simulink model "warp_timer"  (Simulink 7.1)
settings: Solver=ode45  StartTime=0.0  StopTime=1000  RelTol=1e-3
undefined symbols (not defined in the file): gcbh, xlBlockLoadCallback, xlGetSimulinkPeriod
libraries: xbsIndex_r4 x450
(part 2 of 5)

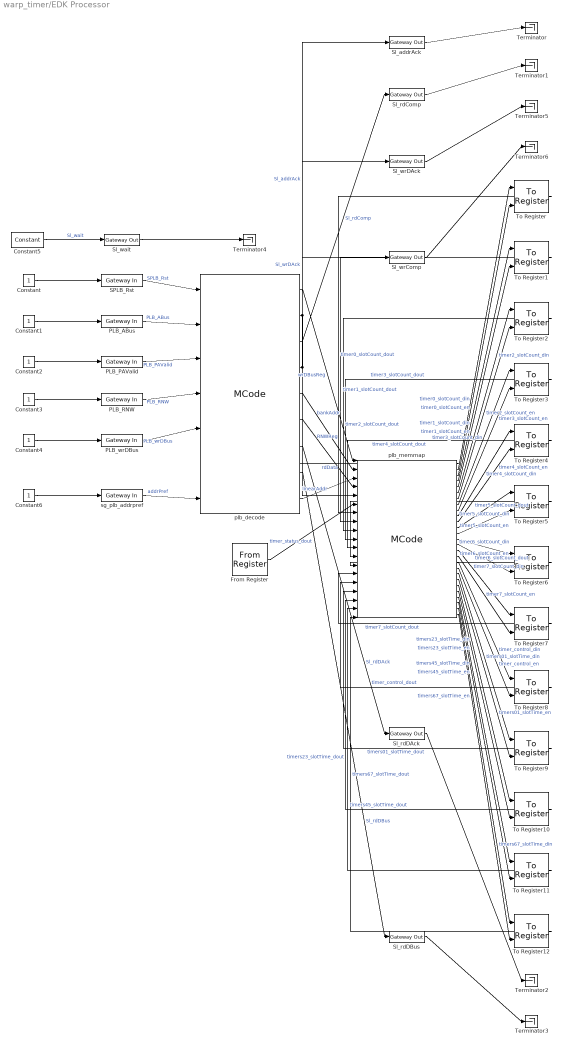
== system warp_timer/EDK Processor ==
  Constant{,1..4,6} (6 alike) : Constant
  Constant5 : xbsIndex_r4/Constant  arith_type=Unsigned  const=0  n_bits=1  bin_pt=0  explicit_period=on  period=xlGetSimulinkPeriod(gcb)  equ=P=C  opselect=C  inp2=PCIN>>17  opr=+  inp1=P  carry=CIN  dbl_ovrd=off  block_type=constant
  From Register : xbsIndex_r4/From Register  shared_memory_name='timer_status'  init=0  period=xlGetSimulinkPeriod(gcb)  ownership=Owned and initialized elsewhere  arith_type=Unsigned  n_bits=32  bin_pt=0  dbl_ovrd=off  block_type=fromreg
      settings: AttributesFormatString=<< %<shared_memory_name> >>  infoedit="Register block that reads data to a shared memory register.  Delay of one sample period."  block_version=10.1.3
  PLB_ABus : xbsIndex_r4/Gateway In  arith_type=Unsigned  n_bits=32  bin_pt=0  quantization="Round  (unbiased: +/- Inf)"  overflow=Saturate  period=xlGetSimulinkPeriod(gcb)  dbl_ovrd=off  timing_constraint=None  locs_specified=off  LOCs={}  block_type=gatewayin
      settings: infoedit="Gateway in block.  Converts inputs of type Simulink integer, double and fixed point to  Xilinx fixed point type.<P><P>Hardware notes:  In hardware these blocks become top level input ports."  sginterface={'Xilinx'=>{'jtaghwcosim'=>{'non_memory_mapped_port'=>'PLB_ABus'}},'iopad'=>{'constraint'=>'#'}}  block_version=10.1.3
  PLB_PAValid : xbsIndex_r4/Gateway In  arith_type=Unsigned  n_bits=1  bin_pt=0  quantization="Round  (unbiased: +/- Inf)"  overflow=Saturate  period=xlGetSimulinkPeriod(gcb)  dbl_ovrd=off  timing_constraint=None  locs_specified=off  LOCs={}  block_type=gatewayin
      settings: infoedit="Gateway in block.  Converts inputs of type Simulink integer, double and fixed point to  Xilinx fixed point type.<P><P>Hardware notes:  In hardware these blocks become top level input ports."  sginterface={'Xilinx'=>{'jtaghwcosim'=>{'non_memory_mapped_port'=>'PLB_PAValid'}},'iopad'=>{'constraint'=>'#'}}  block_version=10.1.3
  PLB_RNW : xbsIndex_r4/Gateway In  arith_type=Unsigned  n_bits=1  bin_pt=0  quantization="Round  (unbiased: +/- Inf)"  overflow=Saturate  period=xlGetSimulinkPeriod(gcb)  dbl_ovrd=off  timing_constraint=None  locs_specified=off  LOCs={}  block_type=gatewayin
      settings: infoedit="Gateway in block.  Converts inputs of type Simulink integer, double and fixed point to  Xilinx fixed point type.<P><P>Hardware notes:  In hardware these blocks become top level input ports."  sginterface={'Xilinx'=>{'jtaghwcosim'=>{'non_memory_mapped_port'=>'PLB_RNW'}},'iopad'=>{'constraint'=>'#'}}  block_version=10.1.3
  PLB_wrDBus : xbsIndex_r4/Gateway In  arith_type=Unsigned  n_bits=32  bin_pt=0  quantization="Round  (unbiased: +/- Inf)"  overflow=Saturate  period=xlGetSimulinkPeriod(gcb)  dbl_ovrd=off  timing_constraint=None  locs_specified=off  LOCs={}  block_type=gatewayin
      settings: infoedit="Gateway in block.  Converts inputs of type Simulink integer, double and fixed point to  Xilinx fixed point type.<P><P>Hardware notes:  In hardware these blocks become top level input ports."  sginterface={'Xilinx'=>{'jtaghwcosim'=>{'non_memory_mapped_port'=>'PLB_wrDBus'}},'iopad'=>{'constraint'=>'#'}}  block_version=10.1.3
  SPLB_Rst : xbsIndex_r4/Gateway In  arith_type=Unsigned  n_bits=1  bin_pt=0  quantization="Round  (unbiased: +/- Inf)"  overflow=Saturate  period=xlGetSimulinkPeriod(gcb)  dbl_ovrd=off  timing_constraint=None  locs_specified=off  LOCs={}  block_type=gatewayin
      settings: infoedit="Gateway in block.  Converts inputs of type Simulink integer, double and fixed point to  Xilinx fixed point type.<P><P>Hardware notes:  In hardware these blocks become top level input ports."  sginterface={'Xilinx'=>{'jtaghwcosim'=>{'non_memory_mapped_port'=>'SPLB_Rst'}},'iopad'=>{'constraint'=>'#'}}  block_version=10.1.3
  Sl_addrAck : xbsIndex_r4/Gateway Out  hdl_port=on  timing_constraint=None  locs_specified=off  LOCs={}  block_type=gatewayout
      settings: infoedit="Gateway out block.  Converts Xilinx fixed point inputs into ouputs of type Simulink integer, double, or fixed point.<P><P>Hardware notes:  In hardware these blocks become top level output ports or are discarded, depending on how they are configured."  sginterface={'Xilinx'=>{'jtaghwcosim'=>{'non_memory_mapped_port'=>'Sl_addrAck'}},'iopad'=>{'constraint'=>'#'}}  block_version=10.1.3
  Sl_rdComp : xbsIndex_r4/Gateway Out  hdl_port=on  timing_constraint=None  locs_specified=off  LOCs={}  block_type=gatewayout
      settings: infoedit="Gateway out block.  Converts Xilinx fixed point inputs into ouputs of type Simulink integer, double, or fixed point.<P><P>Hardware notes:  In hardware these blocks become top level output ports or are discarded, depending on how they are configured."  sginterface={'Xilinx'=>{'jtaghwcosim'=>{'non_memory_mapped_port'=>'Sl_rdComp'}},'iopad'=>{'constraint'=>'#'}}  block_version=10.1.3
  Sl_rdDAck : xbsIndex_r4/Gateway Out  hdl_port=on  timing_constraint=None  locs_specified=off  LOCs={}  block_type=gatewayout
      settings: infoedit="Gateway out block.  Converts Xilinx fixed point inputs into ouputs of type Simulink integer, double, or fixed point.<P><P>Hardware notes:  In hardware these blocks become top level output ports or are discarded, depending on how they are configured."  sginterface={'Xilinx'=>{'jtaghwcosim'=>{'non_memory_mapped_port'=>'Sl_rdDAck'}},'iopad'=>{'constraint'=>'#'}}  block_version=10.1.3
  Sl_rdDBus : xbsIndex_r4/Gateway Out  hdl_port=on  timing_constraint=None  locs_specified=off  LOCs={}  block_type=gatewayout
      settings: infoedit="Gateway out block.  Converts Xilinx fixed point inputs into ouputs of type Simulink integer, double, or fixed point.<P><P>Hardware notes:  In hardware these blocks become top level output ports or are discarded, depending on how they are configured."  sginterface={'Xilinx'=>{'jtaghwcosim'=>{'non_memory_mapped_port'=>'Sl_rdDBus'}},'iopad'=>{'constraint'=>'#'}}  block_version=10.1.3
  Sl_wait : xbsIndex_r4/Gateway Out  hdl_port=on  timing_constraint=None  locs_specified=off  LOCs={}  block_type=gatewayout
      settings: infoedit="Gateway out block.  Converts Xilinx fixed point inputs into ouputs of type Simulink integer, double, or fixed point.<P><P>Hardware notes:  In hardware these blocks become top level output ports or are discarded, depending on how they are configured."  sginterface={'Xilinx'=>{'jtaghwcosim'=>{'non_memory_mapped_port'=>'Sl_wait'}},'iopad'=>{'constraint'=>'#'}}  block_version=10.1.3
  Sl_wrComp : xbsIndex_r4/Gateway Out  hdl_port=on  timing_constraint=None  locs_specified=off  LOCs={}  block_type=gatewayout
      settings: infoedit="Gateway out block.  Converts Xilinx fixed point inputs into ouputs of type Simulink integer, double, or fixed point.<P><P>Hardware notes:  In hardware these blocks become top level output ports or are discarded, depending on how they are configured."  sginterface={'Xilinx'=>{'jtaghwcosim'=>{'non_memory_mapped_port'=>'Sl_wrComp'}},'iopad'=>{'constraint'=>'#'}}  block_version=10.1.3
  Sl_wrDAck : xbsIndex_r4/Gateway Out  hdl_port=on  timing_constraint=None  locs_specified=off  LOCs={}  block_type=gatewayout
      settings: infoedit="Gateway out block.  Converts Xilinx fixed point inputs into ouputs of type Simulink integer, double, or fixed point.<P><P>Hardware notes:  In hardware these blocks become top level output ports or are discarded, depending on how they are configured."  sginterface={'Xilinx'=>{'jtaghwcosim'=>{'non_memory_mapped_port'=>'Sl_wrDAck'}},'iopad'=>{'constraint'=>'#'}}  block_version=10.1.3
  Terminator{,1..6} (7 alike) : Terminator
  To Register : xbsIndex_r4/To Register  shared_memory_name='timer0_slotCount'  init=0  ownership=Owned and initialized elsewhere  explicit_data_type=on  arith_type=Unsigned  n_bits=32  bin_pt=0  dbl_ovrd=off  block_type=toreg
      settings: AttributesFormatString=<< %<shared_memory_name> >>  infoedit="Register block that writes data to a shared memory register.  Delay of one sample period."  block_version=10.1.3
  To Register1 : xbsIndex_r4/To Register  shared_memory_name='timer1_slotCount'  init=0  ownership=Owned and initialized elsewhere  explicit_data_type=on  arith_type=Unsigned  n_bits=32  bin_pt=0  dbl_ovrd=off  block_type=toreg
      settings: AttributesFormatString=<< %<shared_memory_name> >>  infoedit="Register block that writes data to a shared memory register.  Delay of one sample period."  block_version=10.1.3
  To Register10 : xbsIndex_r4/To Register  shared_memory_name='timers23_slotTime'  init=0  ownership=Owned and initialized elsewhere  explicit_data_type=on  arith_type=Unsigned  n_bits=32  bin_pt=0  dbl_ovrd=off  block_type=toreg
      settings: AttributesFormatString=<< %<shared_memory_name> >>  infoedit="Register block that writes data to a shared memory register.  Delay of one sample period."  block_version=10.1.3
  To Register11 : xbsIndex_r4/To Register  shared_memory_name='timers45_slotTime'  init=0  ownership=Owned and initialized elsewhere  explicit_data_type=on  arith_type=Unsigned  n_bits=32  bin_pt=0  dbl_ovrd=off  block_type=toreg
      settings: AttributesFormatString=<< %<shared_memory_name> >>  infoedit="Register block that writes data to a shared memory register.  Delay of one sample period."  block_version=10.1.3
  To Register12 : xbsIndex_r4/To Register  shared_memory_name='timers67_slotTime'  init=0  ownership=Owned and initialized elsewhere  explicit_data_type=on  arith_type=Unsigned  n_bits=32  bin_pt=0  dbl_ovrd=off  block_type=toreg
      settings: AttributesFormatString=<< %<shared_memory_name> >>  infoedit="Register block that writes data to a shared memory register.  Delay of one sample period."  block_version=10.1.3
  To Register2 : xbsIndex_r4/To Register  shared_memory_name='timer2_slotCount'  init=0  ownership=Owned and initialized elsewhere  explicit_data_type=on  arith_type=Unsigned  n_bits=32  bin_pt=0  dbl_ovrd=off  block_type=toreg
      settings: AttributesFormatString=<< %<shared_memory_name> >>  infoedit="Register block that writes data to a shared memory register.  Delay of one sample period."  block_version=10.1.3
  To Register3 : xbsIndex_r4/To Register  shared_memory_name='timer3_slotCount'  init=0  ownership=Owned and initialized elsewhere  explicit_data_type=on  arith_type=Unsigned  n_bits=32  bin_pt=0  dbl_ovrd=off  block_type=toreg
      settings: AttributesFormatString=<< %<shared_memory_name> >>  infoedit="Register block that writes data to a shared memory register.  Delay of one sample period."  block_version=10.1.3
  To Register4 : xbsIndex_r4/To Register  shared_memory_name='timer4_slotCount'  init=0  ownership=Owned and initialized elsewhere  explicit_data_type=on  arith_type=Unsigned  n_bits=32  bin_pt=0  dbl_ovrd=off  block_type=toreg
      settings: AttributesFormatString=<< %<shared_memory_name> >>  infoedit="Register block that writes data to a shared memory register.  Delay of one sample period."  block_version=10.1.3
  To Register5 : xbsIndex_r4/To Register  shared_memory_name='timer5_slotCount'  init=0  ownership=Owned and initialized elsewhere  explicit_data_type=on  arith_type=Unsigned  n_bits=32  bin_pt=0  dbl_ovrd=off  block_type=toreg
      settings: AttributesFormatString=<< %<shared_memory_name> >>  infoedit="Register block that writes data to a shared memory register.  Delay of one sample period."  block_version=10.1.3
  To Register6 : xbsIndex_r4/To Register  shared_memory_name='timer6_slotCount'  init=0  ownership=Owned and initialized elsewhere  explicit_data_type=on  arith_type=Unsigned  n_bits=32  bin_pt=0  dbl_ovrd=off  block_type=toreg
      settings: AttributesFormatString=<< %<shared_memory_name> >>  infoedit="Register block that writes data to a shared memory register.  Delay of one sample period."  block_version=10.1.3
  To Register7 : xbsIndex_r4/To Register  shared_memory_name='timer7_slotCount'  init=0  ownership=Owned and initialized elsewhere  explicit_data_type=on  arith_type=Unsigned  n_bits=32  bin_pt=0  dbl_ovrd=off  block_type=toreg
      settings: AttributesFormatString=<< %<shared_memory_name> >>  infoedit="Register block that writes data to a shared memory register.  Delay of one sample period."  block_version=10.1.3
  To Register8 : xbsIndex_r4/To Register  shared_memory_name='timer_control'  init=0  ownership=Owned and initialized elsewhere  explicit_data_type=on  arith_type=Unsigned  n_bits=32  bin_pt=0  dbl_ovrd=off  block_type=toreg
      settings: AttributesFormatString=<< %<shared_memory_name> >>  infoedit="Register block that writes data to a shared memory register.  Delay of one sample period."  block_version=10.1.3
  To Register9 : xbsIndex_r4/To Register  shared_memory_name='timers01_slotTime'  init=0  ownership=Owned and initialized elsewhere  explicit_data_type=on  arith_type=Unsigned  n_bits=32  bin_pt=0  dbl_ovrd=off  block_type=toreg
      settings: AttributesFormatString=<< %<shared_memory_name> >>  infoedit="Register block that writes data to a shared memory register.  Delay of one sample period."  block_version=10.1.3
  plb_decode : xbsIndex_r4/MCode  mfname=xlmax  explicit_period=off  period=1  dbl_ovrd=off  enable_stdout=off  enable_debug=off  mfilecontent=|  suppress_output=1  defparams={}  hide_port_list={}  block_type=mcode
      | function [wrDBusReg, addrAck, rdComp, wrDAck, bankAddr, RNWReg, rdDAck, rdDBus, linearAddr] = ...
      |     plb_bus_decode(plbRst, plbABus, plbPAValid, plbRNW, plbWrDBus, rdData, addrPref)
      | 
      | % constant variables (TODO: should pass from outside)
      | ADDRPREF_LEN = 20;
      | BANKADDR_LEN = 2;
      | LINEARADDR_LEN = 8;
      | ABUS_LEN = 32;
      | DBUS_LEN = 32;
      | 
      | % declare and initialize persistent variables
      | % register input bus signals
      | persistent plbRstReg_, plbRstReg_ = xl_state(0, {xlBoolean});
      | persistent plbABusReg_, plbABusReg_ = xl_state(0, {xlUnsigned, ABUS_LEN, 0});
      | persistent plbPAValidReg_, plbPAValidReg_ = xl_state(0, {xlBoolean});
      | persistent plbRNWReg_, plbRNWReg_ = xl_state(0, {xlUnsigned, 1, 0});
      | persistent plbWrDBusReg_, plbWrDBusReg_ = xl_state(0, {xlUnsigned, DBUS_LEN, 0});
      | 
      | % ===== rest of the outputs =====
      | 
      | bankAddr   = xl_slice(plbABusReg_, 2+BANKADDR_LEN+LINEARADDR_LEN-1, 2+LINEARADDR_LEN);
      | linearAddr = xl_slice(plbABusReg_, 2+LINEARADDR_LEN-1, 2);
      | RNWReg = plbRNWReg_;
      | wrDBusReg = plbWrDBusReg_;
      | 
      | % ===== p_select =====
      | 
      | % register PAValid
      | persistent aValidReg, aValidReg = xl_state(0, {xlBoolean});
      | aValidReg = plbPAValidReg_;
      | 
      | % extract and register the address prefix
      | addrPref_in = xl_slice(plbABusReg_, xl_nbits(plbABusReg_)-1, xl_nbits(plbABusReg_)-ADDRPREF_LEN);
      | if addrPref_in == addrPref
      |     ps1 = true;
      | else 
      |     ps1 = false;
      | end 
      | 
      | persistent ps1Reg, ps1Reg = xl_state(0, ps1);
      | ps1Reg = ps1;
      | 
      | ps = xl_and(ps1Reg, aValidReg);
      | 
      | % ===== addrAck =====
      | 
      | % register ps
      | persistent psReg, psReg = xl_state(0, ps);
      | 
      | addrAck = xfix({xlUnsigned, 1, 0}, xl_and(xl_not(plbRstReg_), ps, xl_not(psReg)));
      | 
      | psReg = ps;
      | 
      | % ===== rdComp, rd/wr DAck =====
      |  
      | rdComp1 = xfix({xlUnsigned, 1, 0}, xl_and(addrAck, RNWReg));
      | 
      | NUM_rdCompDelay = 3;
      | persistent rdCompDelay, rdCompDelay = xl_state(zeros(1, NUM_rdCompDelay), rdComp1, NUM_rdCompDelay);
      | rdComp2 = rdCompDelay.back;
      | rdCompDelay.push_front_pop_back(rdComp1);
      | 
      | persistent rdCompReg, rdCompReg = xl_state(0, rdComp1);
      | rdComp = rdCompReg;
      | rdCompReg = rdComp2;
      | 
      | persistent rdDAckReg, rdDAckReg = xl_state(0, rdComp1);
      | rdDAck = rdDAckReg;
      | rdDAckReg = rdComp;
      | 
      | persistent wrDAckReg, wrDAckReg = xl_state(0, addrAck);
      | wrDAck = wrDAckReg;
      | wrDAckReg = xl_and(addrAck, xl_not(RNWReg));
      | 
      | % ===== rdDBus =====
      | 
      | rdSel = xl_or(rdComp2, rdComp);
      | 
      | if rdSel == 1
      |     rdDBus1 = rdData;
      | else
      |     rdDBus1 = 0;
      | end % if
      | 
      | persistent rdDBusReg, rdDBusReg = xl_state(0, rdDBus1);
      | rdDBus = rdDBusReg;
      | rdDBusReg = rdDBus1;
      | 
      | % rdDBus = xl_concat(rdDBus32, rdDBus32);
      | % rdDBus = rdDBus32;
      | 
      | % ===== update the persistent variables =====
      | 
      | plbRstReg_ = plbRst;
      | plbABusReg_ = plbABus;
      | plbPAValidReg_ = plbPAValid;
      | plbRNWReg_ = plbRNW;
      | plbWrDBusReg_ = xl_slice(plbWrDBus, DBUS_LEN-1, 0);
      settings: block_version=10.1.3
  plb_memmap : xbsIndex_r4/MCode  mfname=xlmax  explicit_period=off  period=1  dbl_ovrd=off  enable_stdout=off  enable_debug=off  mfilecontent=|  suppress_output=1  defparams={}  hide_port_list={}  block_type=mcode
      | function [read_bank_out, sm_timer0_slotCount_din, sm_timer0_slotCount_en, sm_timer1_slotCount_din, sm_timer1_slotCount_en, sm_timer2_slotCount_din, sm_timer2_slotCount_en, sm_timer3_slotCount_din, sm_timer3_slotCount_en, sm_timer4_slotCount_din, sm_timer4_slotCount_en, sm_timer5_slotCount_din, sm_timer5_slotCount_en, sm_timer6_slotCount_din, sm_timer6_slotCount_en, sm_timer7_slotCount_din, sm_timer7_slotCount_en, sm_timer_control_din, sm_timer_control_en, sm_timers01_slotTime_din, sm_timers01_slotTime_en, sm_timers23_slotTime_din, sm_timers23_slotTime_en, sm_timers45_slotTime_din, sm_timers45_slotTime_en, sm_timers67_slotTime_din, sm_timers67_slotTime_en] = plb_memmap(wrDBus, bankAddr, linearAddr, RNWReg, addrAck, sm_timer_status, sm_timer0_slotCount, sm_timer1_slotCount, sm_timer2_slotCount, sm_timer3_slotCount, sm_timer4_slotCount, sm_timer5_slotCount, sm_timer6_slotCount, sm_timer7_slotCount, sm_timer_control, sm_timers01_slotTime, sm_timers23_slotTime, sm_timers45_slotTime, sm_timers67_slotTime)
      | 
      | 
      | % connvert the input data to UFix_32_0 (the bus data type)
      | % 'From Register' blocks
      | % sm_timer_status_bus = xfix({xlUnsigned, 32, 0}, 0);
      | sm_timer_status_bus = xl_force(sm_timer_status, xlUnsigned, 0);
      | 
      | % 'To Register' blocks
      | 
      | % sm_timer0_slotCount_dout = xfix({xlUnsigned, 32, 0}, 0);
      | sm_timer0_slotCount_dout = xl_force(sm_timer0_slotCount, xlUnsigned, 0);
      | 
      | % sm_timer1_slotCount_dout = xfix({xlUnsigned, 32, 0}, 0);
      | sm_timer1_slotCount_dout = xl_force(sm_timer1_slotCount, xlUnsigned, 0);
      | 
      | % sm_timer2_slotCount_dout = xfix({xlUnsigned, 32, 0}, 0);
      | sm_timer2_slotCount_dout = xl_force(sm_timer2_slotCount, xlUnsigned, 0);
      | 
      | % sm_timer3_slotCount_dout = xfix({xlUnsigned, 32, 0}, 0);
      | sm_timer3_slotCount_dout = xl_force(sm_timer3_slotCount, xlUnsigned, 0);
      | 
      | % sm_timer4_slotCount_dout = xfix({xlUnsigned, 32, 0}, 0);
      | sm_timer4_slotCount_dout = xl_force(sm_timer4_slotCount, xlUnsigned, 0);
      | 
      | % sm_timer5_slotCount_dout = xfix({xlUnsigned, 32, 0}, 0);
      | sm_timer5_slotCount_dout = xl_force(sm_timer5_slotCount, xlUnsigned, 0);
      | 
      | % sm_timer6_slotCount_dout = xfix({xlUnsigned, 32, 0}, 0);
      | sm_timer6_slotCount_dout = xl_force(sm_timer6_slotCount, xlUnsigned, 0);
      | 
      | % sm_timer7_slotCount_dout = xfix({xlUnsigned, 32, 0}, 0);
      | sm_timer7_slotCount_dout = xl_force(sm_timer7_slotCount, xlUnsigned, 0);
      | 
      | % sm_timer_control_dout = xfix({xlUnsigned, 32, 0}, 0);
      | sm_timer_control_dout = xl_force(sm_timer_control, xlUnsigned, 0);
      | 
      | % sm_timers01_slotTime_dout = xfix({xlUnsigned, 32, 0}, 0);
      | sm_timers01_slotTime_dout = xl_force(sm_timers01_slotTime, xlUnsigned, 0);
      | 
      | % sm_timers23_slotTime_dout = xfix({xlUnsigned, 32, 0}, 0);
      | sm_timers23_slotTime_dout = xl_force(sm_timers23_slotTime, xlUnsigned, 0);
      | 
      | % sm_timers45_slotTime_dout = xfix({xlUnsigned, 32, 0}, 0);
      | sm_timers45_slotTime_dout = xl_force(sm_timers45_slotTime, xlUnsigned, 0);
      | 
      | % sm_timers67_slotTime_dout = xfix({xlUnsigned, 32, 0}, 0);
      | sm_timers67_slotTime_dout = xl_force(sm_timers67_slotTime, xlUnsigned, 0);
      | 
      | 
      | % 'From FIFO' blocks
      | % 'To FIFO' blocks
      | % 'Shared Memory' blocks
      | 
      | % 'dout' ports of 'From Register' blocks
      | 
      | % registered register mux output
      | persistent reg_bank_out_reg; reg_bank_out_reg = xl_state(0, {xlUnsigned, 32, 0});
      | reg_bank_out = reg_bank_out_reg;
      | 
      | if linearAddr == 13
      |     reg_bank_out_reg = sm_timer_status_bus;
      | elseif linearAddr == 0
      |     reg_bank_out_reg = sm_timer0_slotCount_dout;
      | elseif linearAddr == 1
      |     reg_bank_out_reg = sm_timer1_slotCount_dout;
      | elseif linearAddr == 2
      |     reg_bank_out_reg = sm_timer2_slotCount_dout;
      | elseif linearAddr == 3
      |     reg_bank_out_reg = sm_timer3_slotCount_dout;
      | elseif linearAddr == 4
      |     reg_bank_out_reg = sm_timer4_slotCount_dout;
      | elseif linearAddr == 5
      |     reg_bank_out_reg = sm_timer5_slotCount_dout;
      | elseif linearAddr == 6
      |     reg_bank_out_reg = sm_timer6_slotCount_dout;
      | elseif linearAddr == 7
      |     reg_bank_out_reg = sm_timer7_slotCount_dout;
      | elseif linearAddr == 8
      |     reg_bank_out_reg = sm_timer_control_dout;
      | elseif linearAddr == 9
      |     reg_bank_out_reg = sm_timers01_slotTime_dout;
      | elseif linearAddr == 10
      |     reg_bank_out_reg = sm_timers23_slotTime_dout;
      | elseif linearAddr == 11
      |     reg_bank_out_reg = sm_timers45_slotTime_dout;
      | elseif linearAddr == 12
      |     reg_bank_out_reg = sm_timers67_slotTime_dout;
      | 
      | end
      | 
      | 
      | % 'From FIFO' and 'To FIFO' blocks
      | 
      | 
      | 
      | 
      | 
      | opCode = xl_concat(addrAck, RNWReg, bankAddr, linearAddr);
      | 
      | % 'Shared Memory' blocks
      | 
      | 
      | 
      | 
      | 
      | % 'din' ports of 'Shared Memory' blocks
      | 
      | 
      | % 'we' ports of 'Shared Memory' blocks
      | 
      | 
      | % 'addr' ports of 'Shared Memory' blocks
      | 
      | 
      | % 're' ports of 'From FIFO' blocks
      | 
      | 
      | % 'en' ports of 'To Register' blocks
      | if opCode == xl_concat(xfix({xlUnsigned, 4, 0}, 10), ...
      |                        xfix({xlUnsigned, xl_nbits(linearAddr), 0}, 0))
      |     sm_timer0_slotCount_en = true;
      | else
      |     sm_timer0_slotCount_en = false;
      | end
      | if opCode == xl_concat(xfix({xlUnsigned, 4, 0}, 10), ...
      |                        xfix({xlUnsigned, xl_nbits(linearAddr), 0}, 1))
      |     sm_timer1_slotCount_en = true;
      | else
      |     sm_timer1_slotCount_en = false;
      | end
      | if opCode == xl_concat(xfix({xlUnsigned, 4, 0}, 10), ...
      |                        xfix({xlUnsigned, xl_nbits(linearAddr), 0}, 2))
      |     sm_timer2_slotCount_en = true;
      | else
      |     sm_timer2_slotCount_en = false;
      | end
      | if opCode == xl_concat(xfix({xlUnsigned, 4, 0}, 10), ...
      |                        xfix({xlUnsigned, xl_nbits(linearAddr), 0}, 3))
      |     sm_timer3_slotCount_en = true;
      | else
      |     sm_timer3_slotCount_en = false;
      | end
      | if opCode == xl_concat(xfix({xlUnsigned, 4, 0}, 10), ...
      |                        xfix({xlUnsigned, xl_nbits(linearAddr), 0}, 4))
      |     sm_timer4_slotCount_en = true;
      | else
      |     sm_timer4_slotCount_en = false;
      | end
      | if opCode == xl_concat(xfix({xlUnsigned, 4, 0}, 10), ...
      |                        xfix({xlUnsigned, xl_nbits(linearAddr), 0}, 5))
      |     sm_timer5_slotCount_en = true;
      | else
      |     sm_timer5_slotCount_en = false;
      | end
      | if opCode == xl_concat(xfix({xlUnsigned, 4, 0}, 10), ...
      |                        xfix({xlUnsigned, xl_nbits(linearAddr), 0}, 6))
      |     sm_timer6_slotCount_en = true;
      | else
      |     sm_timer6_slotCount_en = false;
      | end
      | if opCode == xl_concat(xfix({xlUnsigned, 4, 0}, 10), ...
      |                        xfix({xlUnsigned, xl_nbits(linearAddr), 0}, 7))
      |     sm_timer7_slotCount_en = true;
      | else
      |     sm_timer7_slotCount_en = false;
      | end
      | if opCode == xl_concat(xfix({xlUnsigned, 4, 0}, 10), ...
      |                        xfix({xlUnsigned, xl_nbits(linearAddr), 0}, 8))
      |     sm_timer_control_en = true;
      | else
      |     sm_timer_control_en = false;
      | end
      | if opCode == xl_concat(xfix({xlUnsigned, 4, 0}, 10), ...
      |                        xfix({xlUnsigned, xl_nbits(linearAddr), 0}, 9))
      |     sm_timers01_slotTime_en = true;
      | else
      |     sm_timers01_slotTime_en = false;
      | end
      | if opCode == xl_concat(xfix({xlUnsigned, 4, 0}, 10), ...
      |                        xfix({xlUnsigned, xl_nbits(linearAddr), 0}, 10))
      |     sm_timers23_slotTime_en = true;
      | else
      |     sm_timers23_slotTime_en = false;
      | end
      | if opCode == xl_concat(xfix({xlUnsigned, 4, 0}, 10), ...
      |                        xfix({xlUnsigned, xl_nbits(linearAddr), 0}, 11))
      |     sm_timers45_slotTime_en = true;
      | else
      |     sm_timers45_slotTime_en = false;
      | end
      | if opCode == xl_concat(xfix({xlUnsigned, 4, 0}, 10), ...
      |                        xfix({xlUnsigned, xl_nbits(linearAddr), 0}, 12))
      |     sm_timers67_slotTime_en = true;
      | else
      |     sm_timers67_slotTime_en = false;
      | end
      | 
      | 
      | % 'din' ports of 'To FIFO' blocks
      | 
      | 
      | % 'we' ports of 'To FIFO' blocks
      | 
      | 
      | % 'din' ports of 'To Register' blocks
      | sm_timer0_slotCount_din = xl_force(xl_slice(wrDBus, 32 - 1, 0), ...
      |                                  xlUnsigned, ...
      |                                  0);
      | sm_timer1_slotCount_din = xl_force(xl_slice(wrDBus, 32 - 1, 0), ...
      |                                  xlUnsigned, ...
      |                                  0);
      | sm_timer2_slotCount_din = xl_force(xl_slice(wrDBus, 32 - 1, 0), ...
      |                                  xlUnsigned, ...
      |                                  0);
      | sm_timer3_slotCount_din = xl_force(xl_slice(wrDBus, 32 - 1, 0), ...
      |                                  xlUnsigned, ...
      |                                  0);
      | sm_timer4_slotCount_din = xl_force(xl_slice(wrDBus, 32 - 1, 0), ...
      |                                  xlUnsigned, ...
      |                                  0);
      | sm_timer5_slotCount_din = xl_force(xl_slice(wrDBus, 32 - 1, 0), ...
      |                                  xlUnsigned, ...
      |                                  0);
      | sm_timer6_slotCount_din = xl_force(xl_slice(wrDBus, 32 - 1, 0), ...
      |                                  xlUnsigned, ...
      |                                  0);
      | sm_timer7_slotCount_din = xl_force(xl_slice(wrDBus, 32 - 1, 0), ...
      |                                  xlUnsigned, ...
      |                                  0);
      | sm_timer_control_din = xl_force(xl_slice(wrDBus, 32 - 1, 0), ...
      |                                  xlUnsigned, ...
      |                                  0);
      | sm_timers01_slotTime_din = xl_force(xl_slice(wrDBus, 32 - 1, 0), ...
      |                                  xlUnsigned, ...
      |                                  0);
      | sm_timers23_slotTime_din = xl_force(xl_slice(wrDBus, 32 - 1, 0), ...
      |                                  xlUnsigned, ...
      |                                  0);
      | sm_timers45_slotTime_din = xl_force(xl_slice(wrDBus, 32 - 1, 0), ...
      |                                  xlUnsigned, ...
      |                                  0);
      | sm_timers67_slotTime_din = xl_force(xl_slice(wrDBus, 32 - 1, 0), ...
      |                                  xlUnsigned, ...
      |                                  0);
      | 
      | 
      | persistent read_bank_out_reg; read_bank_out_reg = xl_state(0, {xlUnsigned, 32, 0});
      | read_bank_out = read_bank_out_reg;
      | 
      | persistent bankAddr_reg; bankAddr_reg = xl_state(0, bankAddr);
      | 
      | if bankAddr_reg == 0
      |     % Bank 0: Shared Memories
      |     read_bank_out_reg = 0;
      | elseif bankAddr_reg == 1
      |     % Bank 1: From/To FIFOs
      |     read_bank_out_reg =  0;
      | elseif bankAddr_reg == 2
      |     % Bank 2: From/To Registers
      |     read_bank_out_reg = reg_bank_out;
      | elseif bankAddr_reg == 3
      |     % Bank 3: Configuration Registers
      |     read_bank_out_reg = 0;
      | end
      | 
      | bankAddr_reg = bankAddr;
      settings: block_version=10.1.3
  sg_plb_addrpref : xbsIndex_r4/Gateway In  arith_type=Unsigned  n_bits=20  bin_pt=0  quantization="Round  (unbiased: +/- Inf)"  overflow=Saturate  period=xlGetSimulinkPeriod(gcb)  dbl_ovrd=off  timing_constraint=None  locs_specified=off  LOCs={}  block_type=gatewayin
      settings: infoedit="Gateway in block.  Converts inputs of type Simulink integer, double and fixed point to  Xilinx fixed point type.<P><P>Hardware notes:  In hardware these blocks become top level input ports."  sginterface={'Xilinx'=>{'jtaghwcosim'=>{'non_memory_mapped_port'=>'sg_plb_addrpref'}},'iopad'=>{'constraint'=>'#'}}  block_version=10.1.3
  wires:
  plb_decode/2 -> plb_memmap/5, Sl_addrAck/1  "Sl_addrAck"
  plb_decode/4 -> Sl_wrDAck/1, Sl_wrComp/1  "Sl_wrDAck"
  plb_memmap/27 -> To Register12/2  "timers67_slotTime_en"
  plb_memmap/26 -> To Register12/1  "timers67_slotTime_din"
  plb_memmap/25 -> To Register11/2  "timers45_slotTime_en"
  plb_memmap/24 -> To Register11/1  "timers45_slotTime_din"
  plb_memmap/23 -> To Register10/2  "timers23_slotTime_en"
  plb_memmap/22 -> To Register10/1  "timers23_slotTime_din"
  plb_memmap/21 -> To Register9/2  "timers01_slotTime_en"
  plb_memmap/20 -> To Register9/1  "timers01_slotTime_din"
  plb_memmap/19 -> To Register8/2  "timer_control_en"
  plb_memmap/18 -> To Register8/1  "timer_control_din"
  plb_memmap/17 -> To Register7/2  "timer7_slotCount_en"
  plb_memmap/16 -> To Register7/1  "timer7_slotCount_din"
  plb_memmap/15 -> To Register6/2  "timer6_slotCount_en"
  plb_memmap/14 -> To Register6/1  "timer6_slotCount_din"
  plb_memmap/13 -> To Register5/2  "timer5_slotCount_en"
  plb_memmap/12 -> To Register5/1  "timer5_slotCount_din"
  plb_memmap/11 -> To Register4/2  "timer4_slotCount_en"
  plb_memmap/10 -> To Register4/1  "timer4_slotCount_din"
  plb_memmap/9 -> To Register3/2  "timer3_slotCount_en"
  plb_memmap/8 -> To Register3/1  "timer3_slotCount_din"
  plb_memmap/7 -> To Register2/2  "timer2_slotCount_en"
  plb_memmap/6 -> To Register2/1  "timer2_slotCount_din"
  plb_memmap/5 -> To Register1/2  "timer1_slotCount_en"
  plb_memmap/4 -> To Register1/1  "timer1_slotCount_din"
  plb_memmap/3 -> To Register/2  "timer0_slotCount_en"
  plb_memmap/2 -> To Register/1  "timer0_slotCount_din"
  plb_memmap/1 -> plb_decode/6  "rdData"
  To Register12/1 -> plb_memmap/19  "timers67_slotTime_dout"
  To Register11/1 -> plb_memmap/18  "timers45_slotTime_dout"
  To Register10/1 -> plb_memmap/17  "timers23_slotTime_dout"
  To Register9/1 -> plb_memmap/16  "timers01_slotTime_dout"
  To Register8/1 -> plb_memmap/15  "timer_control_dout"
  To Register7/1 -> plb_memmap/14  "timer7_slotCount_dout"
  To Register6/1 -> plb_memmap/13  "timer6_slotCount_dout"
  To Register5/1 -> plb_memmap/12  "timer5_slotCount_dout"
  To Register4/1 -> plb_memmap/11  "timer4_slotCount_dout"
  To Register3/1 -> plb_memmap/10  "timer3_slotCount_dout"
  To Register2/1 -> plb_memmap/9  "timer2_slotCount_dout"
  To Register1/1 -> plb_memmap/8  "timer1_slotCount_dout"
  To Register/1 -> plb_memmap/7  "timer0_slotCount_dout"
  From Register/1 -> plb_memmap/6  "timer_status_dout"
  plb_decode/6 -> plb_memmap/4  "RNWReg"
  plb_decode/9 -> plb_memmap/3  "linearAddr"
  plb_decode/5 -> plb_memmap/2  "bankAddr"
  plb_decode/1 -> plb_memmap/1  "wrDBusReg"
  plb_decode/8 -> Sl_rdDBus/1  "Sl_rdDBus"
  plb_decode/7 -> Sl_rdDAck/1  "Sl_rdDAck"
  plb_decode/3 -> Sl_rdComp/1  "Sl_rdComp"
  sg_plb_addrpref/1 -> plb_decode/7  "addrPref"
  PLB_wrDBus/1 -> plb_decode/5  "PLB_wrDBus"
  PLB_RNW/1 -> plb_decode/4  "PLB_RNW"
  PLB_PAValid/1 -> plb_decode/3  "PLB_PAValid"
  PLB_ABus/1 -> plb_decode/2  "PLB_ABus"
  SPLB_Rst/1 -> plb_decode/1  "SPLB_Rst"
  Constant6/1 -> sg_plb_addrpref/1
  Constant5/1 -> Sl_wait/1  "Sl_wait"
  Constant4/1 -> PLB_wrDBus/1
  Constant3/1 -> PLB_RNW/1
  Constant2/1 -> PLB_PAValid/1
  Constant1/1 -> PLB_ABus/1
  Constant/1 -> SPLB_Rst/1
  Sl_wrComp/1 -> Terminator6/1
  Sl_wrDAck/1 -> Terminator5/1
  Sl_wait/1 -> Terminator4/1
  Sl_rdDBus/1 -> Terminator3/1
  Sl_rdDAck/1 -> Terminator2/1
  Sl_rdComp/1 -> Terminator1/1
  Sl_addrAck/1 -> Terminator/1

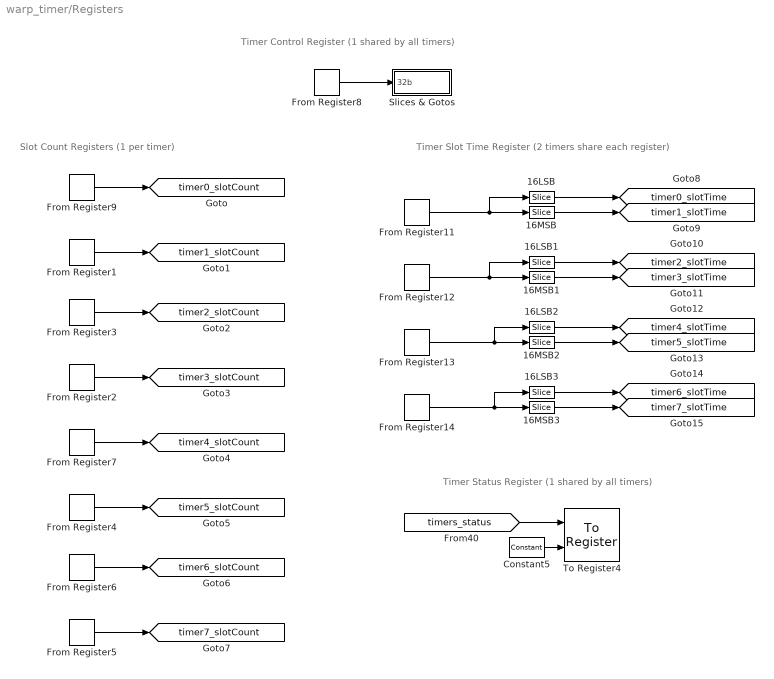
== system warp_timer/Registers ==
  note: Slot Count Registers
      | (1 per timer)
  note: Timer Control Register
      | (1 shared by all timers)
  note: Timer Slot Time Register
      | (2 timers share each register)
  note: Timer Status Register
      | (1 shared by all timers)
  16LSB{,1..3} (4 alike) : xbsIndex_r4/Slice  nbits=16  boolean_output=off  mode=Lower Bit Location + Width  bit1=0  base1=LSB of Input  bit0=0  base0=LSB of Input  dbl_ovrd=off  block_type=slice
      settings: infoedit="Extracts a given range of bits from each input sample and presents it at the output.  The output type is ordinarily unsigned with binary point at zero, but can be Boolean when the slice is one bit wide.<P><P>Hardware notes: In hardware this block costs nothing."  block_version=9.1.01
  16MSB{,1..3} (4 alike) : xbsIndex_r4/Slice  nbits=16  boolean_output=off  mode=Lower Bit Location + Width  bit1=0  base1=LSB of Input  bit0=16  base0=LSB of Input  dbl_ovrd=off  block_type=slice
      settings: infoedit="Extracts a given range of bits from each input sample and presents it at the output.  The output type is ordinarily unsigned with binary point at zero, but can be Boolean when the slice is one bit wide.<P><P>Hardware notes: In hardware this block costs nothing."  block_version=9.1.01
  Constant5 : xbsIndex_r4/Constant  arith_type=Boolean  const=1  n_bits=1  bin_pt=0  explicit_period=off  period=1  equ=P=C  opselect=C  inp2=PCIN>>17  opr=+  inp1=P  carry=CIN  dbl_ovrd=off  block_type=constant
      settings: block_version=8.2
  From Register1 : xbsIndex_r4/From Register  shared_memory_name='timer1_slotCount'  init=500  period=1  ownership=Locally owned and initialized  arith_type=Unsigned  n_bits=32  bin_pt=0  dbl_ovrd=off  block_type=fromreg
      settings: AttributesFormatString=From Register\n<< %<shared_memory_name> >>  infoedit="Register block that reads data to a shared memory register.  Delay of one sample period."  block_version=8.2
  From Register11 : xbsIndex_r4/From Register  shared_memory_name='timers01_slotTime'  init=0  period=1  ownership=Locally owned and initialized  arith_type=Unsigned  n_bits=32  bin_pt=0  dbl_ovrd=off  block_type=fromreg
      settings: AttributesFormatString=From Register\n<< %<shared_memory_name> >>  infoedit="Register block that reads data to a shared memory register.  Delay of one sample period."  block_version=8.2
  From Register12 : xbsIndex_r4/From Register  shared_memory_name='timers23_slotTime'  init=0  period=1  ownership=Locally owned and initialized  arith_type=Unsigned  n_bits=32  bin_pt=0  dbl_ovrd=off  block_type=fromreg
      settings: AttributesFormatString=From Register\n<< %<shared_memory_name> >>  infoedit="Register block that reads data to a shared memory register.  Delay of one sample period."  block_version=8.2
  From Register13 : xbsIndex_r4/From Register  shared_memory_name='timers45_slotTime'  init=0  period=1  ownership=Locally owned and initialized  arith_type=Unsigned  n_bits=32  bin_pt=0  dbl_ovrd=off  block_type=fromreg
      settings: AttributesFormatString=From Register\n<< %<shared_memory_name> >>  infoedit="Register block that reads data to a shared memory register.  Delay of one sample period."  block_version=8.2
  From Register14 : xbsIndex_r4/From Register  shared_memory_name='timers67_slotTime'  init=0  period=1  ownership=Locally owned and initialized  arith_type=Unsigned  n_bits=32  bin_pt=0  dbl_ovrd=off  block_type=fromreg
      settings: AttributesFormatString=From Register\n<< %<shared_memory_name> >>  infoedit="Register block that reads data to a shared memory register.  Delay of one sample period."  block_version=8.2
  From Register2 : xbsIndex_r4/From Register  shared_memory_name='timer3_slotCount'  init=500  period=1  ownership=Locally owned and initialized  arith_type=Unsigned  n_bits=32  bin_pt=0  dbl_ovrd=off  block_type=fromreg
      settings: AttributesFormatString=From Register\n<< %<shared_memory_name> >>  infoedit="Register block that reads data to a shared memory register.  Delay of one sample period."  block_version=8.2
  From Register3 : xbsIndex_r4/From Register  shared_memory_name='timer2_slotCount'  init=500  period=1  ownership=Locally owned and initialized  arith_type=Unsigned  n_bits=32  bin_pt=0  dbl_ovrd=off  block_type=fromreg
      settings: AttributesFormatString=From Register\n<< %<shared_memory_name> >>  infoedit="Register block that reads data to a shared memory register.  Delay of one sample period."  block_version=8.2
  From Register4 : xbsIndex_r4/From Register  shared_memory_name='timer5_slotCount'  init=500  period=1  ownership=Locally owned and initialized  arith_type=Unsigned  n_bits=32  bin_pt=0  dbl_ovrd=off  block_type=fromreg
      settings: AttributesFormatString=From Register\n<< %<shared_memory_name> >>  infoedit="Register block that reads data to a shared memory register.  Delay of one sample period."  block_version=8.2
  From Register5 : xbsIndex_r4/From Register  shared_memory_name='timer7_slotCount'  init=500  period=1  ownership=Locally owned and initialized  arith_type=Unsigned  n_bits=32  bin_pt=0  dbl_ovrd=off  block_type=fromreg
      settings: AttributesFormatString=From Register\n<< %<shared_memory_name> >>  infoedit="Register block that reads data to a shared memory register.  Delay of one sample period."  block_version=8.2
  From Register6 : xbsIndex_r4/From Register  shared_memory_name='timer6_slotCount'  init=500  period=1  ownership=Locally owned and initialized  arith_type=Unsigned  n_bits=32  bin_pt=0  dbl_ovrd=off  block_type=fromreg
      settings: AttributesFormatString=From Register\n<< %<shared_memory_name> >>  infoedit="Register block that reads data to a shared memory register.  Delay of one sample period."  block_version=8.2
  From Register7 : xbsIndex_r4/From Register  shared_memory_name='timer4_slotCount'  init=500  period=1  ownership=Locally owned and initialized  arith_type=Unsigned  n_bits=32  bin_pt=0  dbl_ovrd=off  block_type=fromreg
      settings: AttributesFormatString=From Register\n<< %<shared_memory_name> >>  infoedit="Register block that reads data to a shared memory register.  Delay of one sample period."  block_version=8.2
  From Register8 : xbsIndex_r4/From Register  shared_memory_name='timer_control'  init=0  period=1  ownership=Locally owned and initialized  arith_type=Unsigned  n_bits=32  bin_pt=0  dbl_ovrd=off  block_type=fromreg
      settings: AttributesFormatString=From Register\n<< %<shared_memory_name> >>  infoedit="Register block that reads data to a shared memory register.  Delay of one sample period."  block_version=8.2
  From Register9 : xbsIndex_r4/From Register  shared_memory_name='timer0_slotCount'  init=500  period=1  ownership=Locally owned and initialized  arith_type=Unsigned  n_bits=32  bin_pt=0  dbl_ovrd=off  block_type=fromreg
      settings: AttributesFormatString=From Register\n<< %<shared_memory_name> >>  infoedit="Register block that reads data to a shared memory register.  Delay of one sample period."  block_version=8.2
  Slices & Gotos : Subsystem
  To Register4 : xbsIndex_r4/To Register  shared_memory_name='timer_status'  init=0  ownership=Locally owned and initialized  explicit_data_type=on  arith_type=Unsigned  n_bits=32  bin_pt=0  dbl_ovrd=off  block_type=toreg
      settings: AttributesFormatString=To Register\n<< %<shared_memory_name> >>  infoedit="Register block that writes data to a shared memory register.  Delay of one sample period."  block_version=9.1.01
  tag scope: timer0_slotCount=global, timer0_slotTime=global, timer1_slotCount=global, timer1_slotTime=global, timer2_slotCount=global, timer2_slotTime=global, timer3_slotCount=global, timer3_slotTime=global, timer4_slotCount=global, timer4_slotTime=global, timer5_slotCount=global, timer5_slotTime=global, timer6_slotCount=global, timer6_slotTime=global, timer7_slotCount=global, timer7_slotTime=global
  wires:
  From Register8/1 -> Slices & Gotos/1(32b)
  From Register9/1 -> [timer0_slotCount]
  From Register5/1 -> [timer7_slotCount]
  From Register6/1 -> [timer6_slotCount]
  From Register4/1 -> [timer5_slotCount]
  From Register7/1 -> [timer4_slotCount]
  From Register2/1 -> [timer3_slotCount]
  From Register3/1 -> [timer2_slotCount]
  From Register1/1 -> [timer1_slotCount]
  From Register11/1 -> 16MSB/1, 16LSB/1
  16LSB/1 -> [timer0_slotTime]
  16MSB/1 -> [timer1_slotTime]
  16LSB1/1 -> [timer2_slotTime]
  16MSB1/1 -> [timer3_slotTime]
  16LSB2/1 -> [timer4_slotTime]
  16MSB2/1 -> [timer5_slotTime]
  16LSB3/1 -> [timer6_slotTime]
  16MSB3/1 -> [timer7_slotTime]
  From Register12/1 -> 16LSB1/1, 16MSB1/1
  From Register13/1 -> 16LSB2/1, 16MSB2/1
  From Register14/1 -> 16LSB3/1, 16MSB3/1
  Constant5/1 -> To Register4/2
  [timers_status] -> To Register4/1

== system warp_timer/Status Outputs ==
  T0 : Inport
  T1 : Inport  Port=2
  T2 : Inport  Port=3
  T3 : Inport  Port=4
  T4 : Inport  Port=5
  T5 : Inport  Port=6
  T6 : Inport  Port=7
  T7 : Inport  Port=8
  Concat13 : xbsIndex_r4/Concat  num_inputs=8  dbl_ovrd=off  block_type=concat
      settings: block_version=9.1.01
  LSB+{1..8} (8 alike) : xbsIndex_r4/Slice  nbits=1  boolean_output=off  mode=Lower Bit Location + Width  bit1=0  base1=LSB of Input  bit0=1  base0=LSB of Input  dbl_ovrd=off  block_type=slice
      settings: infoedit="Extracts a given range of bits from each input sample and presents it at the output.  The output type is ordinarily unsigned with binary point at zero, but can be Boolean when the slice is one bit wide.<P><P>Hardware notes: In hardware this block costs nothing."  block_version=9.1.01
  Logical : xbsIndex_r4/Logical  logical_function=OR  inputs=8  en=off  latency=0  precision=Full  arith_type=Unsigned  n_bits=16  bin_pt=0  align_bp=on  dbl_ovrd=off  block_type=logical
  TIMEREXPIRE : xbsIndex_r4/Gateway Out  hdl_port=on  timing_constraint=None  locs_specified=off  LOCs={}  block_type=gatewayout
      settings: infoedit="Gateway out block.  Converts Xilinx fixed point inputs into ouputs of type Simulink integer, double, or fixed point.<P><P>Hardware notes:  In hardware these blocks become top level output ports or are discarded, depending on how they are configured."  block_version=8.2
  timer0_active : xbsIndex_r4/Gateway Out  hdl_port=on  timing_constraint=None  locs_specified=off  LOCs={}  block_type=gatewayout
      settings: infoedit="Gateway out block.  Converts Xilinx fixed point inputs into ouputs of type Simulink integer, double, or fixed point.<P><P>Hardware notes:  In hardware these blocks become top level output ports or are discarded, depending on how they are configured."
  timer1_active : xbsIndex_r4/Gateway Out  hdl_port=on  timing_constraint=None  locs_specified=off  LOCs={}  block_type=gatewayout
      settings: infoedit="Gateway out block.  Converts Xilinx fixed point inputs into ouputs of type Simulink integer, double, or fixed point.<P><P>Hardware notes:  In hardware these blocks become top level output ports or are discarded, depending on how they are configured."
  timer2_active : xbsIndex_r4/Gateway Out  hdl_port=on  timing_constraint=None  locs_specified=off  LOCs={}  block_type=gatewayout
      settings: infoedit="Gateway out block.  Converts Xilinx fixed point inputs into ouputs of type Simulink integer, double, or fixed point.<P><P>Hardware notes:  In hardware these blocks become top level output ports or are discarded, depending on how they are configured."
  timer3_active : xbsIndex_r4/Gateway Out  hdl_port=on  timing_constraint=None  locs_specified=off  LOCs={}  block_type=gatewayout
      settings: infoedit="Gateway out block.  Converts Xilinx fixed point inputs into ouputs of type Simulink integer, double, or fixed point.<P><P>Hardware notes:  In hardware these blocks become top level output ports or are discarded, depending on how they are configured."
  timer4_active : xbsIndex_r4/Gateway Out  hdl_port=on  timing_constraint=None  locs_specified=off  LOCs={}  block_type=gatewayout
      settings: infoedit="Gateway out block.  Converts Xilinx fixed point inputs into ouputs of type Simulink integer, double, or fixed point.<P><P>Hardware notes:  In hardware these blocks become top level output ports or are discarded, depending on how they are configured."
  timer5_active : xbsIndex_r4/Gateway Out  hdl_port=on  timing_constraint=None  locs_specified=off  LOCs={}  block_type=gatewayout
      settings: infoedit="Gateway out block.  Converts Xilinx fixed point inputs into ouputs of type Simulink integer, double, or fixed point.<P><P>Hardware notes:  In hardware these blocks become top level output ports or are discarded, depending on how they are configured."
  timer6_active : xbsIndex_r4/Gateway Out  hdl_port=on  timing_constraint=None  locs_specified=off  LOCs={}  block_type=gatewayout
      settings: infoedit="Gateway out block.  Converts Xilinx fixed point inputs into ouputs of type Simulink integer, double, or fixed point.<P><P>Hardware notes:  In hardware these blocks become top level output ports or are discarded, depending on how they are configured."
  timer7_active : xbsIndex_r4/Gateway Out  hdl_port=on  timing_constraint=None  locs_specified=off  LOCs={}  block_type=gatewayout
      settings: infoedit="Gateway out block.  Converts Xilinx fixed point inputs into ouputs of type Simulink integer, double, or fixed point.<P><P>Hardware notes:  In hardware these blocks become top level output ports or are discarded, depending on how they are configured."
  tag scope: timers_status=global
  wires:
  T7/1 -> Concat13/1, LSB+8/1
  T6/1 -> Concat13/2, LSB+7/1
  T5/1 -> Concat13/3, LSB+6/1
  T4/1 -> Concat13/4, LSB+4/1
  T3/1 -> Concat13/5, LSB+5/1
  T2/1 -> Concat13/6, LSB+3/1
  T1/1 -> Concat13/7, LSB+1/1
  T0/1 -> Concat13/8, LSB+2/1
  LSB+2/1 -> timer0_active/1, Logical/1
  LSB+1/1 -> timer1_active/1, Logical/2
  LSB+3/1 -> timer2_active/1, Logical/3
  LSB+5/1 -> timer3_active/1, Logical/4
  LSB+4/1 -> timer4_active/1, Logical/5
  LSB+6/1 -> timer5_active/1, Logical/6
  LSB+7/1 -> timer6_active/1, Logical/7
  LSB+8/1 -> timer7_active/1, Logical/8
  Logical/1 -> TIMEREXPIRE/1
  Concat13/1 -> [timers_status]
